simulink model "p7_windTurbineModel"  (R2019b)
settings: Solver=ode4  StartTime=0.0  StopTime=TIME_SIM  FixedStep=STEP_SIZE  RelTol=1e-3
values from neighbouring files (symbols this model uses):
  Area = 13069.8108371    [relevantWindTurbineParameters.mat]
  Bd = 6215000    [relevantWindTurbineParameters.mat]
  beta_OP = 0.296705972839    [relevantWindTurbineParameters.mat]
  CP = [0 0 0 0 0 0 0 0.0108523229163 0.0383908516897 0.0728169712581 0.106247295944 0.131224189854 ... (2500 elements, 50x50)]    [relevantWindTurbineParameters.mat]
  Jg = 534.116    [relevantWindTurbineParameters.mat]
  Jr = 59157000    [relevantWindTurbineParameters.mat]
  Kd = 867637000    [relevantWindTurbineParameters.mat]
  Lambda_legend = [0.5 0.948979591837 1.39795918367 1.84693877551 2.29591836735 2.74489795918 3.19387755102 3.64285714286 4.09183673469 4.54081632653 4.98979591837 5.4387755102 ... (50 elements, 50x1)]    [relevantWindTurbineParameters.mat]
  Ng = 97    [relevantWindTurbineParameters.mat]
  Pe_rated = 5000000    [relevantWindTurbineParameters.mat]
  Pitch_legend = [-10 -9.18367346939 -8.36734693878 -7.55102040816 -6.73469387755 -5.91836734694 -5.10204081633 -4.28571428571 -3.4693877551 -2.65306122449 -1.83673469388 -1.02040816327 ... (50 elements, 50x1)]    [relevantWindTurbineParameters.mat]
  R = 64.5    [relevantWindTurbineParameters.mat]
  rho_air = 1.225    [relevantWindTurbineParameters.mat]
  Tg_OP = 40680.3126247    [relevantWindTurbineParameters.mat]
  Ts = 0.05    [relevantWindTurbineParameters.mat]
undefined symbols (not defined in the file or in its folder): CcO, Dd, Ff, Gg, K_FSF, Ki, L, xOP
libraries: simulink_extras x1
settings Model: Creator=Aleks  LastModifiedBy=MSI
settings DataIOCC: ReturnWorkspaceOutputs=off
settings DebuggingCC: ArithmeticOperatorsInVariantConditions=warning
settings SFSimCC: SimUseLocalCustomCode=off  CustomCodeUndefinedFunction=UseInterfaceOnly
settings RTWCC: RTWUseLocalCustomCode=off
settings CodeAppCC: StateflowObjectComments=on

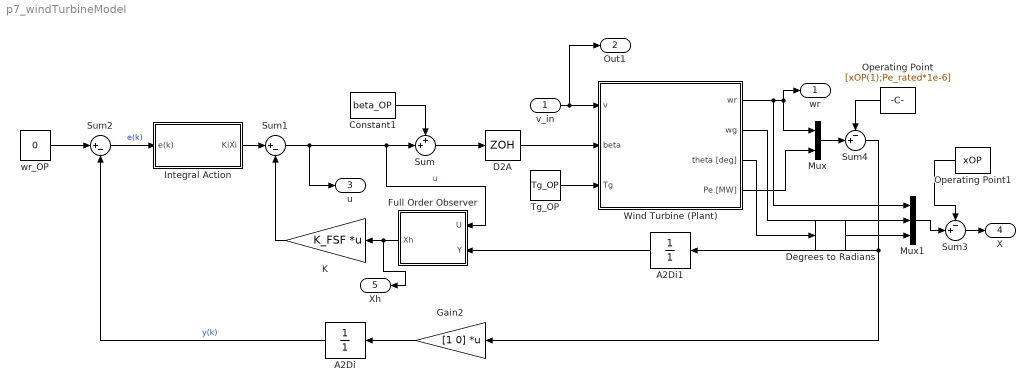
== system p7_windTurbineModel ==
  v_in : Inport
  A2Di : DiscreteTransferFcn  Denominator=[1]  SampleTime=Ts
  A2Di1 : DiscreteTransferFcn  Denominator=[1]  SampleTime=Ts
  Constant1 : Constant  Value=beta_OP  SampleTime=Ts
  D2A : ZeroOrderHold  SampleTime=-1
  Degrees to Radians : simulink_extras/Transformations/Degrees to Radians
  Full Order Observer : Subsystem
  Gain2 : Gain  Gain=[1 0]  Multiplication=Matrix(K*u) (u vector)
  Integral Action : Subsystem
  K : Gain  Gain=K_FSF  Multiplication=Matrix(K*u) (u vector)
  Mux : Mux  Inputs=2
  Mux1 : Mux  Inputs=3
  Operating Point : Constant  Value=[xOP(1);Pe_rated*1e-6]
  Operating Point1 : Constant  Value=xOP
  Sum : Sum  Inputs=++|
  Sum1 : Sum  Inputs=|+-
  Sum2 : Sum  Inputs=|+-
  Sum3 : Sum  Inputs=-+|
  Sum4 : Sum  Inputs=-+|
  Tg_OP : Constant  Value=Tg_OP
  Wind Turbine (Plant) : Subsystem
  wr_OP : Constant  Value=0  SampleTime=Ts
  wr : Outport
  Out1 : Outport  Port=2
  u : Outport  Port=3
  X : Outport  Port=4
  Xh : Outport  Port=5
  wires:
  Tg_OP/1 -> Wind Turbine (Plant)/3(Tg)
  Wind Turbine (Plant)/4(Pe [MW]) -> Mux/2
  Wind Turbine (Plant)/2(wg) -> Mux1/2
  Wind Turbine (Plant)/1(wr) -> Mux1/1, wr/1, Mux/1
  Wind Turbine (Plant)/3(theta [deg]) -> Degrees to Radians/1
  Sum1/1 -> Full Order Observer/1(U), Sum/2, u/1  "u"
  Sum4/1 -> A2Di1/1, Gain2/1
  wr_OP/1 -> Sum2/1
  A2Di/1 -> Sum2/2  "y(k)"
  K/1 -> Sum1/2
  Sum2/1 -> Integral Action/1(e(k))  "e(k)"
  Gain2/1 -> A2Di/1
  Integral Action/1(KiXi) -> Sum1/1
  A2Di1/1 -> Full Order Observer/2(Y)
  Mux/1 -> Sum4/2
  Operating Point/1 -> Sum4/1
  Constant1/1 -> Sum/1
  D2A/1 -> Wind Turbine (Plant)/2(beta)
  Sum/1 -> D2A/1
  v_in/1 -> Out1/1, Wind Turbine (Plant)/1(v)
  Mux1/1 -> Sum3/2
  Operating Point1/1 -> Sum3/1
  Sum3/1 -> X/1
  Full Order Observer/1(Xh) -> Xh/1, K/1
  Degrees to Radians/1 -> Mux1/3

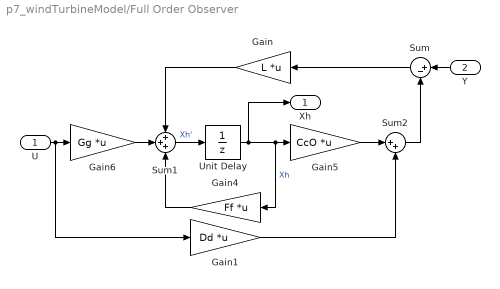
== system p7_windTurbineModel/Full Order Observer ==
  U : Inport
  Y : Inport  Port=2
  Gain : Gain  Gain=L  Multiplication=Matrix(K*u) (u vector)
  Gain1 : Gain  Gain=Dd  Multiplication=Matrix(K*u) (u vector)
  Gain4 : Gain  Gain=Ff  Multiplication=Matrix(K*u) (u vector)
  Gain5 : Gain  Gain=CcO  Multiplication=Matrix(K*u) (u vector)
  Gain6 : Gain  Gain=Gg  Multiplication=Matrix(K*u) (u vector)
  Sum : Sum  Inputs=|+-
  Sum1 : Sum  Inputs=+++
  Sum2 : Sum  Inputs=|++
  Unit Delay : UnitDelay  SampleTime=Ts  HasFrameUpgradeWarning=on
  Xh : Outport
  wires:
  Gain4/1 -> Sum1/3
  Gain6/1 -> Sum1/2
  Sum1/1 -> Unit Delay/1  "Xh'"
  Unit Delay/1 -> Xh/1, Gain4/1, Gain5/1  "Xh"
  U/1 -> Gain1/1, Gain6/1
  Gain/1 -> Sum1/1
  Y/1 -> Sum/1
  Sum/1 -> Gain/1
  Gain1/1 -> Sum2/2
  Gain5/1 -> Sum2/1
  Sum2/1 -> Sum/2

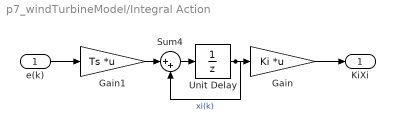
== system p7_windTurbineModel/Integral Action ==
  e(k) : Inport
  Gain : Gain  Gain=Ki  Multiplication=Matrix(K*u) (u vector)
  Gain1 : Gain  Gain=Ts  Multiplication=Matrix(K*u) (u vector)
  Sum4 : Sum  Inputs=|++
  Unit Delay : UnitDelay  SampleTime=Ts  HasFrameUpgradeWarning=on
  KiXi : Outport
  wires:
  Sum4/1 -> Unit Delay/1
  Unit Delay/1 -> Gain/1, Sum4/2  "xi(k)"
  Gain1/1 -> Sum4/1
  e(k)/1 -> Gain1/1
  Gain/1 -> KiXi/1

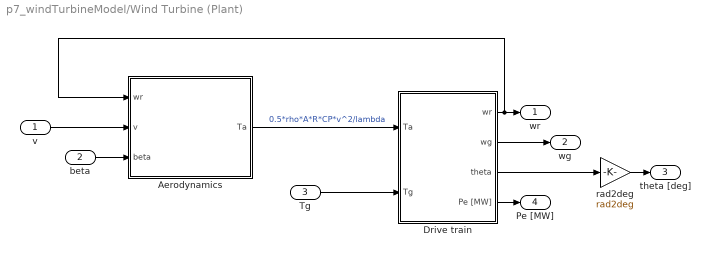
== system p7_windTurbineModel/Wind Turbine (Plant) ==
  v : Inport
  beta : Inport  Port=2
  Tg : Inport  Port=3
  Aerodynamics : Subsystem
  Drive train : Subsystem
  rad2deg : Gain  Gain=rad2deg
  wr : Outport
  wg : Outport  Port=2
  theta [deg] : Outport  Port=3
  Pe [MW] : Outport  Port=4
  wires:
  beta/1 -> Aerodynamics/3(beta)
  v/1 -> Aerodynamics/2(v)
  Aerodynamics/1(Ta) -> Drive train/1(Ta)  "0.5*rho*A*R*CP*v^2/lambda"
  Tg/1 -> Drive train/2(Tg)
  Drive train/3(theta) -> rad2deg/1
  Drive train/1(wr) -> Aerodynamics/1(wr), wr/1
  Drive train/2(wg) -> wg/1
  rad2deg/1 -> theta [deg]/1
  Drive train/4(Pe [MW]) -> Pe [MW]/1

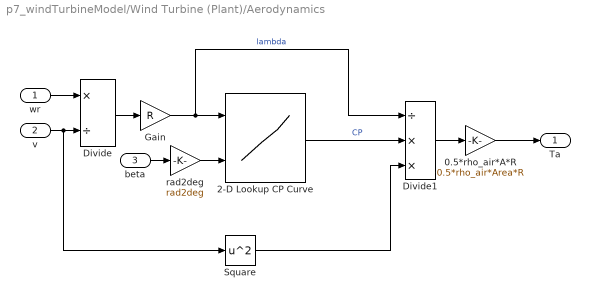
== system p7_windTurbineModel/Wind Turbine (Plant)/Aerodynamics ==
  wr : Inport
  v : Inport  Port=2
  beta : Inport  Port=3
  0.5*rho_air*A*R : Gain  Gain=0.5*rho_air*Area*R
  2-D Lookup CP Curve : Lookup_n-D  BreakpointsForDimension1=Lambda_legend  BreakpointsForDimension2=Pitch_legend  Table=CP  InternalRulePriority=Speed  RndMeth=Simplest  InputSameDT=on
  Divide : Product  Inputs=*/
  Divide1 : Product  Inputs=/**
  Gain : Gain  Gain=R
  Square : Math  Operator=square  SaturateOnIntegerOverflow=on
  rad2deg : Gain  Gain=rad2deg
  Ta : Outport
  wires:
  v/1 -> Square/1, Divide/2
  wr/1 -> Divide/1
  Divide/1 -> Gain/1
  Gain/1 -> Divide1/1, 2-D Lookup CP Curve/1  "lambda"
  rad2deg/1 -> 2-D Lookup CP Curve/2
  beta/1 -> rad2deg/1
  2-D Lookup CP Curve/1 -> Divide1/2  "CP"
  Square/1 -> Divide1/3
  Divide1/1 -> 0.5*rho_air*A*R/1
  0.5*rho_air*A*R/1 -> Ta/1

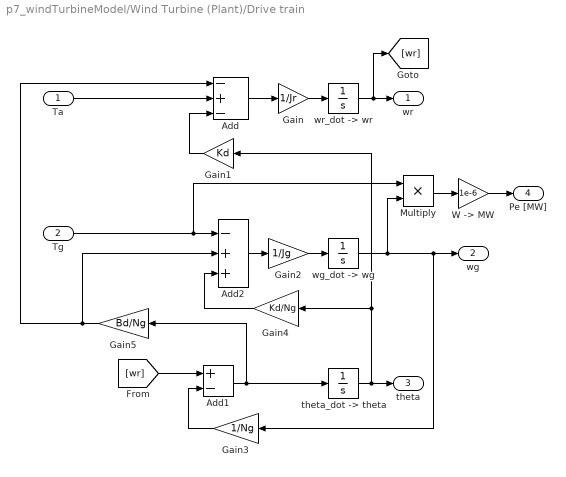
== system p7_windTurbineModel/Wind Turbine (Plant)/Drive train ==
  Ta : Inport
  Tg : Inport  Port=2
  Add : Sum  Inputs=-+-
  Add1 : Sum  Inputs=+-
  Add2 : Sum  Inputs=-++
  Gain : Gain  Gain=1/Jr
  Gain1 : Gain  Gain=Kd
  Gain2 : Gain  Gain=1/Jg
  Gain3 : Gain  Gain=1/Ng
  Gain4 : Gain  Gain=Kd/Ng
  Gain5 : Gain  Gain=Bd/Ng
  Multiply : Product
  "W -> MW" : Gain  Gain=1e-6
  "theta_dot -> theta" : Integrator  Priority=3  InitialCondition=xOP(3)
  "wg_dot -> wg" : Integrator  Priority=2  InitialCondition=xOP(2)
  "wr_dot -> wr" : Integrator  Priority=1  InitialCondition=xOP(1)
  wr : Outport
  wg : Outport  Port=2
  theta : Outport  Port=3
  Pe [MW] : Outport  Port=4
  wires:
  Gain/1 -> "wr_dot -> wr"/1
  "wr_dot -> wr"/1 -> [wr], wr/1
  Add/1 -> Gain/1
  Ta/1 -> Add/2
  Gain1/1 -> Add/3
  Gain2/1 -> "wg_dot -> wg"/1
  "wg_dot -> wg"/1 -> Multiply/2, wg/1, Gain3/1
  "theta_dot -> theta"/1 -> Gain4/1, Gain1/1, theta/1
  Add1/1 -> Gain5/1, "theta_dot -> theta"/1
  [wr] -> Add1/1
  Gain3/1 -> Add1/2
  Add2/1 -> Gain2/1
  Gain4/1 -> Add2/3
  Tg/1 -> Multiply/1, Add2/1
  Gain5/1 -> Add2/2, Add/1
  Multiply/1 -> "W -> MW"/1
  "W -> MW"/1 -> Pe [MW]/1
